simulink model "FullCardioLabModel"  (R2023b)
settings: Solver=FixedStepDiscrete  StartTime=0.0  StopTime=param_sim_time  FixedStep=1/fs  MaxStep=1/fs  RelTol=1e-3
undefined symbols (not defined in the file): analyses, fdesignblkfcn, fs, gcbh, param_tot_samples
libraries: dspstat3 x13, SCGAnalysis_SignalGenerationLib x2
(part 7 of 20)

== system FullCardioLabModel/SCG Preprocessing/Enabled SCG Preprocessing Subsystem/Filtfiltering/Bandpass Filter 1 ==
  In : Inport
  Generated Filter Block : DiscreteFir  Tag=BlockMethodSubSystem  Coefficients=[-0.00978480817658140822 0.00796999512757773539 0.00147001916949499392 -0.00206976963634824965 -0.00243890991203668658 -0.000924134149516313568 0.000721734906667209327 0.00129711475091750009 0.00065625391365372091 -0.000505332991407668681 -0.00128012722911580298 -0.00118584056106419973 -0.00039637962604269618 0.000462570629013598245 0.000795239340671749051 0.000413152706796936372 -0.000373518377931796681 -0.00101662167067725949 -0.00109601261216089613 -0.000593906547901142264 0.000134350294683468992 0.000600271945192584993 0.000514574052205236292 -5.24294882567629715e-05 -0.000721006732066104515 -0.00106936812683964427 -0.000885784329197715666 -0.000306368867509999767 0.000299921121108523685 0.000550903008052714251 0.000305129539031473278 -0.000280348626868086933 -0.000834835852167923817 -0.00102988416243433227 -0.000749730060180390395 -0.000183844427687669172 0.000330781953284103988 0.00047445671354907936 0.000187158515118488676 -0.000375706516283815298 -0.000841441599320367052 -0.000980583400495469836 -0.000677521760008548222 -0.000143136714861160914 0.000296905261906706748 0.000427455994316721874 0.000136983215127181666 -0.000377779512804672765 -0.000807928899011784254 -0.000914634913298793578 -0.000653887485439136069 -0.000162386642358197084 0.000270410746944849676 0.000394818020750986717 0.000144292032000489871 -0.000318126126834031081 -0.000730717848546076263 -0.00086298202242188508 -0.00064618322535159073 -0.000197068691395557781 0.000227657437070462456 0.000390339376956013893 0.000202019386220474471 -0.000218262841065602572 -0.000630398467645967419 -0.00080203368163468756 -0.000643386601296825722 -0.000239583998883380767 0.000186056910795609053 0.000403403846244415891 0.000291609858585218675 -8.0073200147873241e-05 -0.000501540638877883077 -0.000730203151560260776 -0.000640276523076389989 -0.000277375534437485863 0.000156493764593555848 0.000431561395434954648 0.000397367103231406095 8.29189622613074411e-05 -0.000340599175797020681 -0.000631305624859729254 -0.000622947681400656383 -0.000317342453510103845 0.000133455335091095105 0.000471287365521899941 0.000526528964861475179 0.000266844016988344239 -0.0001601129539922299 -0.000507941523151899982 -0.000580953412745202537 -0.000334693556591638395 0.000109719501490277742 0.00051336064834933649 0.000657877410861215997 0.000469632889522447717 5.66691264263484711e-05 -0.000351746005523791172 -0.000520266671699537702 -0.000342073082938880945 9.47970697973939325e-05 0.000556210436752843543 0.000795382016377059399 0.000685450046797950164 0.00028975233342428677 -0.000168394924182673438 -0.000424984820321507441 -0.000326854493346978461 8.34347145895603635e-05 0.000590237414229426551 0.000924037851917057789 0.000905501272636722405 0.000546953829290874557 5.01002670601818621e-05 -0.000300380671440419263 -0.000297252550696250231 7.24448185069438358e-05 0.000616892125762856145 0.00104469796439651363 0.00112540106874017593 0.000815941579190881928 0.000293722454277331739 -0.000147131313195209023 -0.000243553418517207927 6.68821353141186079e-05 0.000631331563724703911 0.00114457781901174073 0.00133020230521633132 0.00109202570585962395 0.000561661563460189397 4.12191178191870775e-05 -0.00016882560370949873 6.18472916976157343e-05 0.00062369924511362885 0.00121794150913751985 0.00152009478062344614 0.00136753539574503095 0.000847811546794769366 0.00025306973421013602 -7.61054743152740051e-05 5.94169316982789947e-05 0.00059970992777688345 0.0012585684356427357 0.00167936422330930207 0.00163112458376199823 0.0011411690442859185 0.000486071978403059717 3.87954501415224492e-05 5.99888187074658106e-05 0.000552926215868729926 0.00125934973898137446 0.00179616995776501727 0.00186851973153338131 0.00143595292525264023 0.000740124310155090728 0.000171789154675156572 5.8420326905926699e-05 0.000478305096295866404 0.00121446318353980232 0.00186532763417885153 0.00207320507044296944 0.00171914297636405005 0.00100075009001191558 0.000316849149569703372 5.78099051731434589e-05 ...(+13949 chars)]  InputProcessing=Columns as channels (frame based)
  Out : Outport  VectorParamsAs1DForOutWhenUnconnected=off
  wires:
  Generated Filter Block/1 -> Out/1
  In/1 -> Generated Filter Block/1

== system FullCardioLabModel/SCG Preprocessing/Enabled SCG Preprocessing Subsystem/Filtfiltering/Bandpass Filter 2 ==
  In : Inport
  Generated Filter Block : DiscreteFir  Tag=BlockMethodSubSystem  Coefficients=[-0.00978480817658140822 0.00796999512757773539 0.00147001916949499392 -0.00206976963634824965 -0.00243890991203668658 -0.000924134149516313568 0.000721734906667209327 0.00129711475091750009 0.00065625391365372091 -0.000505332991407668681 -0.00128012722911580298 -0.00118584056106419973 -0.00039637962604269618 0.000462570629013598245 0.000795239340671749051 0.000413152706796936372 -0.000373518377931796681 -0.00101662167067725949 -0.00109601261216089613 -0.000593906547901142264 0.000134350294683468992 0.000600271945192584993 0.000514574052205236292 -5.24294882567629715e-05 -0.000721006732066104515 -0.00106936812683964427 -0.000885784329197715666 -0.000306368867509999767 0.000299921121108523685 0.000550903008052714251 0.000305129539031473278 -0.000280348626868086933 -0.000834835852167923817 -0.00102988416243433227 -0.000749730060180390395 -0.000183844427687669172 0.000330781953284103988 0.00047445671354907936 0.000187158515118488676 -0.000375706516283815298 -0.000841441599320367052 -0.000980583400495469836 -0.000677521760008548222 -0.000143136714861160914 0.000296905261906706748 0.000427455994316721874 0.000136983215127181666 -0.000377779512804672765 -0.000807928899011784254 -0.000914634913298793578 -0.000653887485439136069 -0.000162386642358197084 0.000270410746944849676 0.000394818020750986717 0.000144292032000489871 -0.000318126126834031081 -0.000730717848546076263 -0.00086298202242188508 -0.00064618322535159073 -0.000197068691395557781 0.000227657437070462456 0.000390339376956013893 0.000202019386220474471 -0.000218262841065602572 -0.000630398467645967419 -0.00080203368163468756 -0.000643386601296825722 -0.000239583998883380767 0.000186056910795609053 0.000403403846244415891 0.000291609858585218675 -8.0073200147873241e-05 -0.000501540638877883077 -0.000730203151560260776 -0.000640276523076389989 -0.000277375534437485863 0.000156493764593555848 0.000431561395434954648 0.000397367103231406095 8.29189622613074411e-05 -0.000340599175797020681 -0.000631305624859729254 -0.000622947681400656383 -0.000317342453510103845 0.000133455335091095105 0.000471287365521899941 0.000526528964861475179 0.000266844016988344239 -0.0001601129539922299 -0.000507941523151899982 -0.000580953412745202537 -0.000334693556591638395 0.000109719501490277742 0.00051336064834933649 0.000657877410861215997 0.000469632889522447717 5.66691264263484711e-05 -0.000351746005523791172 -0.000520266671699537702 -0.000342073082938880945 9.47970697973939325e-05 0.000556210436752843543 0.000795382016377059399 0.000685450046797950164 0.00028975233342428677 -0.000168394924182673438 -0.000424984820321507441 -0.000326854493346978461 8.34347145895603635e-05 0.000590237414229426551 0.000924037851917057789 0.000905501272636722405 0.000546953829290874557 5.01002670601818621e-05 -0.000300380671440419263 -0.000297252550696250231 7.24448185069438358e-05 0.000616892125762856145 0.00104469796439651363 0.00112540106874017593 0.000815941579190881928 0.000293722454277331739 -0.000147131313195209023 -0.000243553418517207927 6.68821353141186079e-05 0.000631331563724703911 0.00114457781901174073 0.00133020230521633132 0.00109202570585962395 0.000561661563460189397 4.12191178191870775e-05 -0.00016882560370949873 6.18472916976157343e-05 0.00062369924511362885 0.00121794150913751985 0.00152009478062344614 0.00136753539574503095 0.000847811546794769366 0.00025306973421013602 -7.61054743152740051e-05 5.94169316982789947e-05 0.00059970992777688345 0.0012585684356427357 0.00167936422330930207 0.00163112458376199823 0.0011411690442859185 0.000486071978403059717 3.87954501415224492e-05 5.99888187074658106e-05 0.000552926215868729926 0.00125934973898137446 0.00179616995776501727 0.00186851973153338131 0.00143595292525264023 0.000740124310155090728 0.000171789154675156572 5.8420326905926699e-05 0.000478305096295866404 0.00121446318353980232 0.00186532763417885153 0.00207320507044296944 0.00171914297636405005 0.00100075009001191558 0.000316849149569703372 5.78099051731434589e-05 ...(+13949 chars)]  InputProcessing=Columns as channels (frame based)
  Out : Outport  VectorParamsAs1DForOutWhenUnconnected=off
  wires:
  In/1 -> Generated Filter Block/1
  Generated Filter Block/1 -> Out/1

== system FullCardioLabModel/SCG Preprocessing/Enabled SCG Preprocessing Subsystem/To Workspace: Processed SCGxyz/To Workspace SCG Enabled Subsystem ==
  note: The subsystem is only enabled when it receives a (non-zero) signal
  In1 : Inport
  Enable : EnablePort
  To Workspace SCG : ToWorkspace  VariableName=out_scg_xyz_preprocessing  SaveFormat=Structure  SampleTime=-1
  wires:
  In1/1 -> To Workspace SCG/1

== system FullCardioLabModel/SCG Analysis/Enabled SCG Analysis Subsystem/3D Anisotropy Characterization/Average Cycle Max Diameter//Volume Calculator/SCG xyz Average Cycle ==
  in_ecg_r : Inport
  in_scg_xyz : Inport  Port=2
  Average SCGxyz Cycle Calculator : MATLAB Function  TreatAsAtomicUnit=on
  Constant : Constant
  Fixed-Size Converter 2 : Selector  NumberOfDimensions=2  IndexOptions=Starting and ending indices (port),Index vector (dialog)  Indices=[1:min(analyses.ecg.RR)],[1 2 3]  OutputSizes=1,1
  Min RR Calculator : MATLAB Function  TreatAsAtomicUnit=on
  Mux : Mux  Inputs=2
  out_scg_xyz_avgcycle : Outport  VectorParamsAs1DForOutWhenUnconnected=off
  wires:
  in_scg_xyz/1 -> Average SCGxyz Cycle Calculator/2(scgxyz)
  in_ecg_r/1 -> Min RR Calculator/1(r_pos), Average SCGxyz Cycle Calculator/1(r_pos)
  Average SCGxyz Cycle Calculator/1(scgxyz_avgcycle) -> Fixed-Size Converter 2/1
  Fixed-Size Converter 2/1 -> out_scg_xyz_avgcycle/1
  Constant/1 -> Mux/1
  Min RR Calculator/1(min_rr) -> Mux/2
  Mux/1 -> Fixed-Size Converter 2/2

== system FullCardioLabModel/SCG Analysis/Enabled SCG Analysis Subsystem/3D Anisotropy Characterization/Average Cycle Max//Median Diameter Calculator/SCG xyz Average Cycle ==
  in_ecg_r : Inport
  in_scg_xyz : Inport  Port=2
  Average SCGxyz Cycle Calculator : MATLAB Function  TreatAsAtomicUnit=on
  Constant : Constant
  Fixed-Size Converter 2 : Selector  NumberOfDimensions=2  IndexOptions=Starting and ending indices (port),Index vector (dialog)  Indices=[1:min(analyses.ecg.RR)],[1 2 3]  OutputSizes=1,1
  Min RR Calculator : MATLAB Function  TreatAsAtomicUnit=on
  Mux : Mux  Inputs=2
  out_scg_xyz_avgcycle : Outport  VectorParamsAs1DForOutWhenUnconnected=off
  wires:
  in_scg_xyz/1 -> Average SCGxyz Cycle Calculator/2(scgxyz)
  in_ecg_r/1 -> Min RR Calculator/1(r_pos), Average SCGxyz Cycle Calculator/1(r_pos)
  Average SCGxyz Cycle Calculator/1(scgxyz_avgcycle) -> Fixed-Size Converter 2/1
  Fixed-Size Converter 2/1 -> out_scg_xyz_avgcycle/1
  Constant/1 -> Mux/1
  Min RR Calculator/1(min_rr) -> Mux/2
  Mux/1 -> Fixed-Size Converter 2/2

== system FullCardioLabModel/SCG Analysis/Enabled SCG Analysis Subsystem/All Signals Signal Metric Characterization/SCG 2D Mod Signal Metric Characterization/Average Cycle-to-cycle Morphological Variability Calculator ==
  note: This subsystem is only enabled when its signal metric flag is raised.
  in_r_pos : Inport
  in_scg_signal : Inport  Port=2
  Enable : EnablePort
  Average Cycle-to-cycle Morphological Variability Calculator : MATLAB Function  TreatAsAtomicUnit=on
  Constant : Constant  Value=fs
  out_morphological_variability : Outport
  wires:
  Constant/1 -> Average Cycle-to-cycle Morphological Variability Calculator/1(fs)
  Average Cycle-to-cycle Morphological Variability Calculator/1(variability) -> out_morphological_variability/1
  in_scg_signal/1 -> Average Cycle-to-cycle Morphological Variability Calculator/3(scg_signal)
  in_r_pos/1 -> Average Cycle-to-cycle Morphological Variability Calculator/2(r_pos)

== system FullCardioLabModel/SCG Analysis/Enabled SCG Analysis Subsystem/All Signals Signal Metric Characterization/SCG 2D Mod Signal Metric Characterization/Average S1 peak-to-peak Amplitude Calculator ==
  note: This subsystem is only enabled when its signal metric flag is raised.
  in_r_pos : Inport
  in_scg_sig : Inport  Port=2
  Enable : EnablePort
  Average S1p2p Amplitude Calculator : MATLAB Function  TreatAsAtomicUnit=on
  Constant : Constant  Value=fs
  out_average_s1p2pamp : Outport
  wires:
  Constant/1 -> Average S1p2p Amplitude Calculator/1(fs)
  in_r_pos/1 -> Average S1p2p Amplitude Calculator/2(r_pos)
  Average S1p2p Amplitude Calculator/1(average_s1p2pamp) -> out_average_s1p2pamp/1
  in_scg_sig/1 -> Average S1p2p Amplitude Calculator/3(scg_signal)

== system FullCardioLabModel/SCG Analysis/Enabled SCG Analysis Subsystem/All Signals Signal Metric Characterization/SCG 2D Mod Signal Metric Characterization/Average S2 peak-to-peak Amplitude Calculator ==
  note: This subsystem is only enabled when its signal metric flag is raised.
  in_r_pos : Inport
  in_scg_signal : Inport  Port=2
  Enable : EnablePort
  Average S2p2p Amplitude Calculator : MATLAB Function  TreatAsAtomicUnit=on
  Constant : Constant  Value=fs
  out_scg_signal_average_s2p2pamp : Outport
  wires:
  in_scg_signal/1 -> Average S2p2p Amplitude Calculator/3(scg_signal)
  Average S2p2p Amplitude Calculator/1(average_s2p2pamp) -> out_scg_signal_average_s2p2pamp/1
  in_r_pos/1 -> Average S2p2p Amplitude Calculator/2(r_pos)
  Constant/1 -> Average S2p2p Amplitude Calculator/1(fs)

== system FullCardioLabModel/SCG Analysis/Enabled SCG Analysis Subsystem/All Signals Signal Metric Characterization/SCG 2D Mod Signal Metric Characterization/Average Signal-to-Noise Ratio Calculator ==
  note: This subsystem is only enabled when its signal metric flag is raised.
  in_r_pos : Inport
  in_scg_signal : Inport  Port=2
  Enable : EnablePort  PropagateVarSize=During execution
  Average S1 Signal-to-Noise Ratio : Subsystem
  Average S1X Signal-to-Noise Ratio : Subsystem
  Average S2 Signal-to-Noise Ratio : Subsystem
  Average S2X Signal-to-Noise Ratio : Subsystem
  out_scg_signal_average_s1snr : Outport
  out_scg_signal_average_s1Xsnr : Outport  Port=2
  out_scg_signal_average_s2snr : Outport  Port=3
  out_scg_signal_average_s2Xsnr : Outport  Port=4
  wires:
  Average S2X Signal-to-Noise Ratio/1(average_s2Xsnr) -> out_scg_signal_average_s2Xsnr/1
  in_r_pos/1 -> Average S1 Signal-to-Noise Ratio/1(r_pos), Average S2X Signal-to-Noise Ratio/1(r_pos), Average S2 Signal-to-Noise Ratio/1(r_pos), Average S1X Signal-to-Noise Ratio/1(r_pos)
  Average S2 Signal-to-Noise Ratio/1(average_s2snr) -> out_scg_signal_average_s2snr/1
  Average S1X Signal-to-Noise Ratio/1(average_s1Xsnr) -> out_scg_signal_average_s1Xsnr/1
  in_scg_signal/1 -> Average S2X Signal-to-Noise Ratio/2(scg_signal), Average S2 Signal-to-Noise Ratio/2(scg_signal), Average S1X Signal-to-Noise Ratio/2(scg_signal), Average S1 Signal-to-Noise Ratio/2(scg_signal)
  Average S1 Signal-to-Noise Ratio/1(average_s1snr) -> out_scg_signal_average_s1snr/1

== system FullCardioLabModel/SCG Analysis/Enabled SCG Analysis Subsystem/All Signals Signal Metric Characterization/SCG 2D Mod Signal Metric Characterization/Spectral Distribution Calculator ==
  note: This subsystem is only enabled when its signal metric flag is raised.
  in_r_pos : Inport
  in_scg_signal : Inport  Port=2
  Enable : EnablePort
  Constant : Constant  Value=fs
  Constant1 : Constant  Value=entire_cycle
  Constant2 : Constant  Value=s1
  Constant3 : Constant  Value=s2
  Constant4 : Constant  Value=f_band_lo
  Constant5 : Constant  Value=f_band_mid
  Constant6 : Constant  Value=f_band_hi
  Spectral Distribution Calculator : MATLAB Function  TreatAsAtomicUnit=on
  out_entire_cycle_spectral_distribution : Outport
  out_s1_spectral_distribution : Outport  Port=2
  out_s2_spectral_distribution : Outport  Port=3
  wires:
  in_r_pos/1 -> Spectral Distribution Calculator/2(r_pos)
  in_scg_signal/1 -> Spectral Distribution Calculator/3(scg_signal)
  Spectral Distribution Calculator/1(entire_cycle_nsd) -> out_entire_cycle_spectral_distribution/1
  Constant/1 -> Spectral Distribution Calculator/1(fs)
  Constant1/1 -> Spectral Distribution Calculator/4(entire_cycle_flag)
  Constant4/1 -> Spectral Distribution Calculator/7(f_band_lo)
  Constant6/1 -> Spectral Distribution Calculator/9(f_band_hi)
  Constant5/1 -> Spectral Distribution Calculator/8(f_band_mid)
  Constant3/1 -> Spectral Distribution Calculator/6(s2_flag)
  Constant2/1 -> Spectral Distribution Calculator/5(s1_flag)
  Spectral Distribution Calculator/3(s2_nsd) -> out_s2_spectral_distribution/1
  Spectral Distribution Calculator/2(s1_nsd) -> out_s1_spectral_distribution/1

== system FullCardioLabModel/SCG Analysis/Enabled SCG Analysis Subsystem/All Signals Signal Metric Characterization/SCG 2D Mod Signal Metric Characterization/Variance ==
  note: This subsystem is only enabled when its signal metric flag is raised.
  in_scg_signal : Inport
  Enable : EnablePort
  Variance : dspstat3/Variance  run=off  InputProcessing=Columns as channels (frame based)  reset_popup=None  directionMode=Each column  dimension=1  roiEnable=off  roiType=Rectangles  roiPortion=Entire ROI  roiOutput=Individual statistics for each ROI  roiFlag=off  roundingMode=Floor  overflowMode=off
  out_scg_signal_var : Outport
  wires:
  Variance/1 -> out_scg_signal_var/1
  in_scg_signal/1 -> Variance/1

== system FullCardioLabModel/SCG Analysis/Enabled SCG Analysis Subsystem/All Signals Signal Metric Characterization/SCG 3D Mod Signal Metric Characterization/Average Cycle-to-cycle Morphological Variability Calculator ==
  note: This subsystem is only enabled when its signal metric flag is raised.
  in_r_pos : Inport
  in_scg_signal : Inport  Port=2
  Enable : EnablePort
  Average Cycle-to-cycle Morphological Variability Calculator : MATLAB Function  TreatAsAtomicUnit=on
  Constant : Constant  Value=fs
  out_morphological_variability : Outport
  wires:
  in_r_pos/1 -> Average Cycle-to-cycle Morphological Variability Calculator/2(r_pos)
  in_scg_signal/1 -> Average Cycle-to-cycle Morphological Variability Calculator/3(scg_signal)
  Average Cycle-to-cycle Morphological Variability Calculator/1(variability) -> out_morphological_variability/1
  Constant/1 -> Average Cycle-to-cycle Morphological Variability Calculator/1(fs)

== system FullCardioLabModel/SCG Analysis/Enabled SCG Analysis Subsystem/All Signals Signal Metric Characterization/SCG 3D Mod Signal Metric Characterization/Average S1 peak-to-peak Amplitude Calculator ==
  note: This subsystem is only enabled when its signal metric flag is raised.
  in_r_pos : Inport
  in_scg_sig : Inport  Port=2
  Enable : EnablePort
  Average S1p2p Amplitude Calculator : MATLAB Function  TreatAsAtomicUnit=on
  Constant : Constant  Value=fs
  out_average_s1p2pamp : Outport
  wires:
  in_scg_sig/1 -> Average S1p2p Amplitude Calculator/3(scg_signal)
  Average S1p2p Amplitude Calculator/1(average_s1p2pamp) -> out_average_s1p2pamp/1
  in_r_pos/1 -> Average S1p2p Amplitude Calculator/2(r_pos)
  Constant/1 -> Average S1p2p Amplitude Calculator/1(fs)

== system FullCardioLabModel/SCG Analysis/Enabled SCG Analysis Subsystem/All Signals Signal Metric Characterization/SCG 3D Mod Signal Metric Characterization/Average S2 peak-to-peak Amplitude Calculator ==
  note: This subsystem is only enabled when its signal metric flag is raised.
  in_r_pos : Inport
  in_scg_signal : Inport  Port=2
  Enable : EnablePort
  Average S2p2p Amplitude Calculator : MATLAB Function  TreatAsAtomicUnit=on
  Constant : Constant  Value=fs
  out_scg_signal_average_s2p2pamp : Outport
  wires:
  Constant/1 -> Average S2p2p Amplitude Calculator/1(fs)
  in_r_pos/1 -> Average S2p2p Amplitude Calculator/2(r_pos)
  Average S2p2p Amplitude Calculator/1(average_s2p2pamp) -> out_scg_signal_average_s2p2pamp/1
  in_scg_signal/1 -> Average S2p2p Amplitude Calculator/3(scg_signal)

== system FullCardioLabModel/SCG Analysis/Enabled SCG Analysis Subsystem/All Signals Signal Metric Characterization/SCG 3D Mod Signal Metric Characterization/Average Signal-to-Noise Ratio Calculator ==
  note: This subsystem is only enabled when its signal metric flag is raised.
  in_r_pos : Inport
  in_scg_signal : Inport  Port=2
  Enable : EnablePort  PropagateVarSize=During execution
  Average S1 Signal-to-Noise Ratio : Subsystem
  Average S1X Signal-to-Noise Ratio : Subsystem
  Average S2 Signal-to-Noise Ratio : Subsystem
  Average S2X Signal-to-Noise Ratio : Subsystem
  out_scg_signal_average_s1snr : Outport
  out_scg_signal_average_s1Xsnr : Outport  Port=2
  out_scg_signal_average_s2snr : Outport  Port=3
  out_scg_signal_average_s2Xsnr : Outport  Port=4
  wires:
  Average S1 Signal-to-Noise Ratio/1(average_s1snr) -> out_scg_signal_average_s1snr/1
  in_scg_signal/1 -> Average S1 Signal-to-Noise Ratio/2(scg_signal), Average S1X Signal-to-Noise Ratio/2(scg_signal), Average S2 Signal-to-Noise Ratio/2(scg_signal), Average S2X Signal-to-Noise Ratio/2(scg_signal)
  Average S1X Signal-to-Noise Ratio/1(average_s1Xsnr) -> out_scg_signal_average_s1Xsnr/1
  Average S2 Signal-to-Noise Ratio/1(average_s2snr) -> out_scg_signal_average_s2snr/1
  in_r_pos/1 -> Average S1X Signal-to-Noise Ratio/1(r_pos), Average S2 Signal-to-Noise Ratio/1(r_pos), Average S2X Signal-to-Noise Ratio/1(r_pos), Average S1 Signal-to-Noise Ratio/1(r_pos)
  Average S2X Signal-to-Noise Ratio/1(average_s2Xsnr) -> out_scg_signal_average_s2Xsnr/1
